simulink model "obstacleAvoidance"  (R2024b)
settings: Solver=VariableStepAuto  StartTime=0.0  StopTime=5  RelTol=1e-3
values from neighbouring files (symbols this model uses):
  TimeStep = 0.02    [obstacleAvoidance_data.sldd]
undefined symbols (not defined in the file or in its folder): driving, x0
libraries: drivingscenarioandsensors x2, simulink_extras x1
settings Model: DataDictionary=obstacleAvoidance_data.sldd  PacingRate=0.500000  Creator=kiwamoto  LastModifiedBy=tshintai
settings OptimizationCC: DefaultParameterBehavior=Inlined  EnhancedBackFolding=on  PassReuseOutputArgsAs=Individual arguments  ZeroExternalMemoryAtStartup=off  ZeroInternalMemoryAtStartup=off  OptimizeBlockOrder=speed  DifferentSizesBufferReuse=on  OptimizationCustomize=off  EfficientTunableParamExpr=on
settings DebuggingCC: ParameterTunabilityLossMsg=error  UnconnectedInputMsg=warning  UnconnectedOutputMsg=warning  UnconnectedLineMsg=warning
settings ModelReferenceCC: EnableRefExpFcnMdlSchedulingChecks=on
settings SFSimCC: MATLABDynamicMemAlloc=off
settings RTWCC: Description=Embedded Coder  SystemTargetFile=ert.tlc  TemplateMakefile=ert_default_tmf  CodeExecutionProfiling=on  CodeProfilingSaveOptions=AllData  GPUComputeCapability=3.5  DLArmComputeVersion=19.05
settings CodeAppCC: ForceParamTrailComments=on  IgnoreCustomStorageClasses=off  OperatorAnnotations=on  SimulinkDataObjDesc=on  SFDataObjDesc=on  InsertBlockDesc=on
settings ERTTargetCC: TargetLangStandard=C99 (ISO)  GenerateSampleERTMain=on  ERTCustomFileTemplate=example_file_process.tlc  DynamicArrayContainerType=coder::array

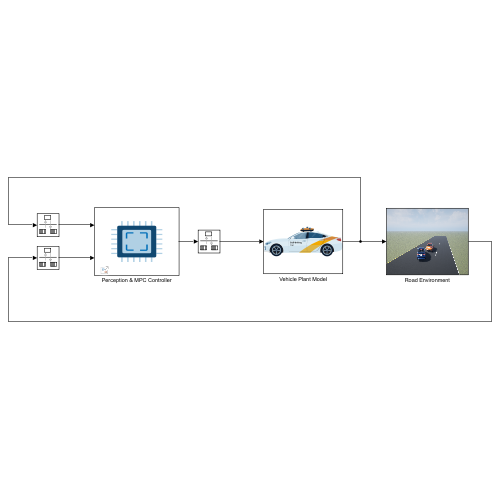
[thumbnail: Simulink's stored preview of the top-level diagram]
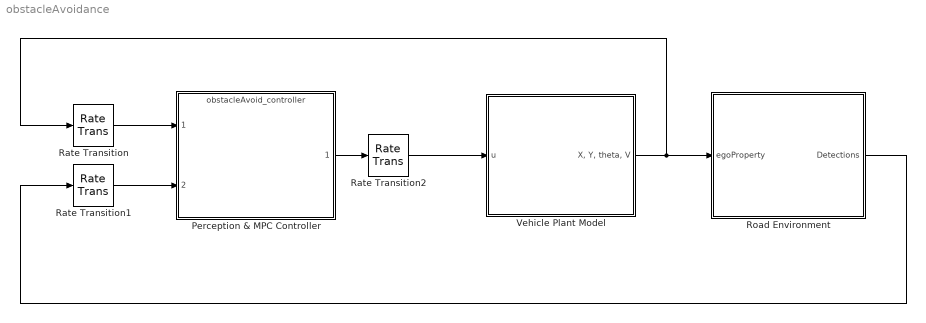
== system obstacleAvoidance ==
  Perception & MPC Controller : ModelReference  ModelNameDialog=obstacleAvoid_controller.slx  SimulationMode=Normal  ModelReferenceVersion=8.0
      mask Display: image('cpu-chip.svg'); % Use "Edit Image" on toolstrip to change.
  Rate Transition : RateTransition  OutPortSampleTime=TimeStep
  Rate Transition1 : RateTransition  OutPortSampleTime=TimeStep
  Rate Transition2 : RateTransition
  Road Environment : Subsystem
      mask Display: image('environment.PNG'); % Use "Edit Image" on toolstrip to change.
  Vehicle Plant Model : Subsystem
      mask Display: image('self-driving-car.svg'); % Use "Edit Image" on toolstrip to change.
  wires:
  Vehicle Plant Model/1("X, Y, theta, V") -> Rate Transition/1, Road Environment/1(egoProperty)
  Perception & MPC Controller/1 -> Rate Transition2/1
  Road Environment/1(Detections) -> Rate Transition1/1
  Rate Transition/1 -> Perception & MPC Controller/1
  Rate Transition1/1 -> Perception & MPC Controller/2
  Rate Transition2/1 -> Vehicle Plant Model/1(u)

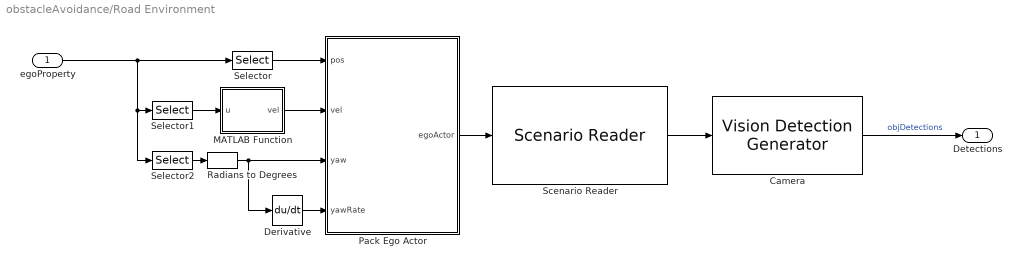
== system obstacleAvoidance/Road Environment ==
  egoProperty : Inport
  Camera : drivingscenarioandsensors/Vision Detection Generator  SensorIndex=1  DetectorOutput=Objects only  UpdateInterval=TimeStep  LaneUpdateInterval=TimeStep  SensorLocation=[3.7 0]  Height=1.1  Yaw=0  Pitch=0  Roll=0  BusNameSource=Auto  BusName=BusObjectDetections  BusName2Source=Auto  BusName2=BusLaneDetections  MaxNumDetectionsSource=Property  MaxNumDetections=1  MaxNumLanesSource=Property  MaxNumLanes=30  DetectionCoordinates=Sensor Cartesian  SimulateUsing=Interpreted execution  MaxRange=DetectionDistance  BoundingBoxAccuracy=10  ProcessNoiseIntensity=2  MaxSpeed=50  MaxAllowedOcclusion=0.2  MinObjectImageSize=[15 15]  DetectionProbability=1  FalsePositivesPerImage=0  MinLaneImageSize=[1 1]  LaneBoundaryAccuracy=1  HasNoise=off  InitialSeedSource=Repeatable  InitialSeed=0  UsedSeed=0  ActorProfilesSource=From Scenario Reader block  ActorProfilesParameters=driving.internal.ActorProfilesParameters  ActorProfilesExpression=[struct('ActorID',1,'ClassID',1,'Length',5,'Width',2,'Height',1.4,'OriginOffset',[-1.5 0 0],'MeshVertices',[4 1 0.857439446366782;4 -1 0.857439446366782;4 -1 0.314878892733564;4 1 0.314878892733564;4 1 0.857439446366782;2.75 1 0.993079584775086;2.75 -1 0.993079584775086;4 -1 0.857439446366782;2 0.8 1.4;0.5 0.8 1.4;0.5 -0.8 1.4;2 -0.8 1.4;-0.25 1 0.993079584775086;-1 1 0.857439446366782;-1 -1 0.857439446366782;-0.25 -1 0.993079584775086;4 1 0.857439446366782;4 1 0.314878892733564;2.75 1 0.314878892733564;2.75 1 0.993079584775086;2.75 1 0.993079584775086;2.75 1 0.314878892733564;-0.25 1 0.314878892733564;-0.25 1 0.993079584775086;-0.25 1 0.993079584775086;-0.25 1 0.314878892733564;-1 1 0.355570934256055;-1 1 0.857439446366782;2.75 1 0.993079584775086;-0.25 1 0.993079584775086;0.5 0.8 1.4;2 0.8 1.4;4 -1 0.857439446366782;4 -1 0.314878892733564;2.75 -1 0.314878892733564;2.75 -1 0.993079584775086;2.75 -1 0.993079584775086;2.75 -1 0.314878892733564;-0.25 -1 0.314878892733564;-0.25 -1 0.993079584775086;-0.25 -1 0.993079584775086;-0.25 -1 0.314878892733564;-1 -1 0.355570934256055;-1 -1 0.857439446366782;2.75 -1 0.993079584775086;-0.25 -1 0.993079584775086;0.5 -0.8 1.4;2 -0.8 1.4;-0.25 1 0.993079584775086;-0.25 -1 0.993079584775086;0.5 -0.8 1.4;0.5 0.8 1.4;2.75 -1 0.993079584775086;2 -0.8 1.4;2 0.8 1.4;2.75 1 0.993079584775086;-1 1 0.857439446366782;-1 1 0.355570934256055;-1 -1 0.355570934256055;-1 -1 0.857439446366782;4 1 0.314878892733564;4 -1 0.314878892733564;-0.25 -1 0.314878892733564;-0.25 1 0.314878892733564;-0.25 1 0.314878892733564;-1 1 0.355570934256055;-1 -1 0.355570934256055;-0.25 -1 0.314878892733564;0.0638297872340425 -0.7 0;0.0638297872340425 -0.966666666666667 0;0.267053411696866 -0.7 0.0601365173421445;0.267053411696866 -0.966666666666667 0.0601365173421445;0.392652518931835 -0.7 0.217575963708927;0.392652518931835 -0.966666666666667 0.217575963708927;0.392652518931835 -0.7 0.412181821758201;0.392652518931835 -0.966666666666667 0.412181821758201;0.267053411696866 -0.7 0.569621268124983;0.267053411696866 -0.966666666666667 0.569621268124983;0.0638297872340425 -0.7 0.629757785467128;0.0638297872340425 -0.966666666666667 0.629757785467128;-0.139393837228781 -0.7 0.569621268124983;-0.139393837228781 -0.966666666666667 0.569621268124983;-0.26499294446375 -0.7 0.412181821758201;-0.26499294446375 -0.966666666666667 0.412181821758201;-0.26499294446375 -0.7 0.217575963708927;-0.26499294446375 -0.966666666666667 0.217575963708927;-0.139393837228781 -0.7 0.0601365173421445;-0.139393837228781 -0.966666666666667 0.0601365173421445;0.0638297872340425 -0.7 0;0.0638297872340425 -0.966666666666667 0;0.0638297872340425 -0.7 0;0.267053411696866 -0.7 0.0601365173421445;0.392652518931835 -0.7 0.217575963708927;0.392652518931835 -0.7 0.412181821758201;0.267053411696866 -0.7 0.569621268124983;0.0638297872340425 -0.7 0.629757785467128;-0.139393837228781 -0.7 0.569621268124983;-0.26499294446375 -0.7 0.412181821758201;-0.26499294446375 -0.7 0.217575963708927;-0.139393837228781 -0.7 0.0601365173421445;0.0638297872340425 -0.966666666666667 0;0.267053411696866 -0.966666666666667 0.0601365173421445;0.392652518931835 -0.966666666666667 0.217575963708927;0.392652518931835 -0.966666666666667 0.412181821758201;0.267053411696866 -0.966666666666667 0.569621268124983;0.0638297872340425 -0.966666666666667 0.629757785467128;-0.139393837228781 -0.966666666666667 0.569621268124983;-0.26499294446375 -0.966666666666667 0.412181821758201;-0.26499294446375 -0.966666666666667 0.217575963708927;-0.139393837228781 -0.966666666666667 0.0601365173421445;0.0638297872340425 0.966666666666667 0;0.0638297872340425 0.7 0;0.267053411696866 0.966666666666667 0.0601365173421445;0.267053411696866 0.7 0.0601365173421445;0.392652518931835 0.966666666666667 0.217575963708927;0.392652518931835 0.7 0.217575963708927;0.392652518931835 0.966666666666667 0.412181821758201;0.392652518931835 0.7 0.412181821758201;0.267053411696866 0.966666666666667 0.569621268124983;0.267053411696866 0.7 0.569621268124983;0.0638297872340425 0.966666666666667 0.629757785467128;0.0638297872340425 0.7 ...(+5114 chars)],'MeshFaces',[1 2 3;3 4 1;5 6 7;7 8 5;9 10 11;11 12 9;13 14 15;15 16 13;17 18 19;19 20 17;21 22 23;23 24 21;25 26 27;27 28 25;29 30 31;31 32 29;33 34 35;35 36 33;37 38 39;39 40 37;41 42 43;43 44 41;45 46 47;47 48 45;49 50 51;51 52 49;53 54 55;55 56 53;57 58 59;59 60 57;61 62 63;63 64 61;65 66 67;67 68 65;69 71 72;72 70 69;71 73 74;74 72 71;73 75 76;76 74 73;75 77 78;78 76 75;77 79 80;80 78 77;79 81 82;82 80 79;81 83 84;84 82 81;83 85 86;86 84 83;85 87 88;88 86 85;87 89 90;90 88 87;91 92 93;91 93 94;91 94 95;91 95 96;91 96 97;91 97 98;91 98 99;91 99 100;101 102 103;101 103 104;101 104 105;101 105 106;101 106 107;101 107 108;101 108 109;101 109 110;111 113 114;114 112 111;113 115 116;116 114 113;115 117 118;118 116 115;117 119 120;120 118 117;119 121 122;122 120 119;121 123 124;124 122 121;123 125 126;126 124 123;125 127 128;128 126 125;127 129 130;130 128 127;129 131 132;132 130 129;133 134 135;133 135 136;133 136 137;133 137 138;133 138 139;133 139 140;133 140 141;133 141 142;143 144 145;143 145 146;143 146 147;143 147 148;143 148 149;143 149 150;143 150 151;143 151 152;153 155 156;156 154 153;155 157 158;158 156 155;157 159 160;160 158 157;159 161 162;162 160 159;161 163 164;164 162 161;163 165 166;166 164 163;165 167 168;168 166 165;167 169 170;170 168 167;169 171 172;172 170 169;171 173 174;174 172 171;175 176 177;175 177 178;175 178 179;175 179 180;175 180 181;175 181 182;175 182 183;175 183 184;185 186 187;185 187 188;185 188 189;185 189 190;185 190 191;185 191 192;185 192 193;185 193 194;195 197 198;198 196 195;197 199 200;200 198 197;199 201 202;202 200 199;201 203 204;204 202 201;203 205 206;206 204 203;205 207 208;208 206 205;207 209 210;210 208 207;209 211 212;212 210 209;211 213 214;214 212 211;213 215 216;216 214 213;217 218 219;217 219 220;217 220 221;217 221 222;217 222 223;217 223 224;217 224 225;217 225 226;227 228 229;227 229 230;227 230 231;227 231 232;227 232 233;227 233 234;227 234 235;227 235 236],'RCSPattern',[10 10;10 10],'RCSAzimuthAngles',[-180 180],'RCSElevationAngles',[-90 90]); struct('ActorID',2,'ClassID',1,'Length',5,'Width',2,'Height',1.4,'OriginOffset',[-1.5 0 0],'MeshVertices',[4 1 0.857439446366782;4 -1 0.857439446366782;4 -1 0.314878892733564;4 1 0.314878892733564;4 1 0.857439446366782;2.75 1 0.993079584775086;2.75 -1 0.993079584775086;4 -1 0.857439446366782;2 0.8 1.4;0.5 0.8 1.4;0.5 -0.8 1.4;2 -0.8 1.4;-0.25 1 0.993079584775086;-1 1 0.857439446366782;-1 -1 0.857439446366782;-0.25 -1 0.993079584775086;4 1 0.857439446366782;4 1 0.314878892733564;2.75 1 0.314878892733564;2.75 1 0.993079584775086;2.75 1 0.993079584775086;2.75 1 0.314878892733564;-0.25 1 0.314878892733564;-0.25 1 0.993079584775086;-0.25 1 0.993079584775086;-0.25 1 0.314878892733564;-1 1 0.355570934256055;-1 1 0.857439446366782;2.75 1 0.993079584775086;-0.25 1 0.993079584775086;0.5 0.8 1.4;2 0.8 1.4;4 -1 0.857439446366782;4 -1 0.314878892733564;2.75 -1 0.314878892733564;2.75 -1 0.993079584775086;2.75 -1 0.993079584775086;2.75 -1 0.314878892733564;-0.25 -1 0.314878892733564;-0.25 -1 0.993079584775086;-0.25 -1 0.993079584775086;-0.25 -1 0.314878892733564;-1 -1 0.355570934256055;-1 -1 0.857439446366782;2.75 -1 0.993079584775086;-0.25 -1 0.993079584775086;0.5 -0.8 1.4;2 -0.8 1.4;-0.25 1 0.993079584775086;-0.25 -1 0.993079584775086;0.5 -0.8 1.4;0.5 0.8 1.4;2.75 -1 0.993079584775086;2 -0.8 1.4;2 0.8 1.4;2.75 1 0.993079584775086;-1 1 0.857439446366782;-1 1 0.355570934256055;-1 -1 0.355570934256055;-1 -1 0.857439446366782;4 1 0.314878892733564;4 -1 0.314878892733564;-0.25 -1 0.314878892733564;-0.25 1 0.314878892733564;-0.25 1 0.314878892733564;-1 1 0.355570934256055;-1 -1 0.355570934256055;-0.25 -1 0.314878892733564;0.0638297872340425 -0.7 0;0.0638297872340425 -0.966666666666667 0;0.267053411696866 -0.7 0.0601365173421445;0.267053411696866 -0.966666666666667 0.0601365173421445;0.392652518931835 -0.7 0.217575963708927;0.392652518931835 -0.966666666666667 0.217575963708927;0.392652518931835 -0.7 0.412181821758201;0.392652518931835 -0.966666666666667 0.412181821758201;0.267053411696866 -0.7 0.569621268124983;0.267053411696866 -0.966666666666667 0.569621268124983;0.0638297872340425 -0.7 0.629757785467128;0.0638297872340425 -0.966666666666667 0.629757785467128;-0.139393837228781 -0.7 0.569621268124983;-0.139393837228781 -0.966666666666667 0.569621268124983;-0.26499294446375 -0.7 0.412181821758201;-0.26499294446375 -0.966666666666667 0.412181821758201;-0.26499294446375 -0.7 0.217575963708927;-0.26499294446375 -0.966666666666667 0.217575963708927;-0.139393837228781 -0.7 0.0601365173421445;-0.139393837228781 -0.966666666666667 0.0601365173421445;0.0638297872340425 -0.7 0;0.0638297872340425 -0.966666666666667 0;0.0638297872340425 -0.7 0;0.267053411696866 -0.7 0.0601365173421445;0.392652518931835 -0.7 0.217575963708927;0.392652518931835 -0.7 0.412181821758201;0.267053411696866 -0.7 0.569621268124983;0.0638297872340425 -0.7 0.629757785467128;-0.139393837228781 -0.7 0.569621268124983;-0.26499294446375 -0.7 0.412181821758201;-0.26499294446375 -0.7 0.217575963708927;-0.139393837228781 -0.7 0.0601365173421445;0.0638297872340425 -0.966666666666667 0;0.267053411696866 -0.966666666666667 0.0601365173421445;0.392652518931835 -0.966666666666667 0.217575963708927;0.392652518931835 -0.966666666666667 0.412181821758201;0.267053411696866 -0.966666666666667 0.569621268124983;0.0638297872340425 -0.966666666666667 0.629757785467128;-0.139393837228781 -0.966666666666667 0.569621268124983;-0.26499294446375 -0.966666666666667 0.412181821758201;-0.26499294446375 -0.966666666666667 0.217575963708927;-0.139393837228781 -0.966666666666667 0.0601365173421445;0.0638297872340425 0.966666666666667 0;0.0638297872340425 0.7 0;0.267053411696866 0.966666666666667 0.0601365173421445;0.267053411696866 0.7 0.0601365173421445;0.392652518931835 0.966666666666667 0.217575963708927;0.392652518931835 0.7 0.217575963708927;0.392652518931835 0.966666666666667 0.412181821758201;0.392652518931835 0.7 0.412181821758201;0.267053411696866 0.966666666666667 0.569621268124983;0.267053411696866 0.7 0.569621268124983;0.0638297872340425 0.966666666666667 0.629757785467128;0.0638297872340425 0.7 ...(+5114 chars)],'MeshFaces',[1 2 3;3 4 1;5 6 7;7 8 5;9 10 11;11 12 9;13 14 15;15 16 13;17 18 19;19 20 17;21 22 23;23 24 21;25 26 27;27 28 25;29 30 31;31 32 29;33 34 35;35 36 33;37 38 39;39 40 37;41 42 43;43 44 41;45 46 47;47 48 45;49 50 51;51 52 49;53 54 55;55 56 53;57 58 59;59 60 57;61 62 63;63 64 61;65 66 67;67 68 65;69 71 72;72 70 69;71 73 74;74 72 71;73 75 76;76 74 73;75 77 78;78 76 75;77 79 80;80 78 77;79 81 82;82 80 79;81 83 84;84 82 81;83 85 86;86 84 83;85 87 88;88 86 85;87 89 90;90 88 87;91 92 93;91 93 94;91 94 95;91 95 96;91 96 97;91 97 98;91 98 99;91 99 100;101 102 103;101 103 104;101 104 105;101 105 106;101 106 107;101 107 108;101 108 109;101 109 110;111 113 114;114 112 111;113 115 116;116 114 113;115 117 118;118 116 115;117 119 120;120 118 117;119 121 122;122 120 119;121 123 124;124 122 121;123 125 126;126 124 123;125 127 128;128 126 125;127 129 130;130 128 127;129 131 132;132 130 129;133 134 135;133 135 136;133 136 137;133 137 138;133 138 139;133 139 140;133 140 141;133 141 142;143 144 145;143 145 146;143 146 147;143 147 148;143 148 149;143 149 150;143 150 151;143 151 152;153 155 156;156 154 153;155 157 158;158 156 155;157 159 160;160 158 157;159 161 162;162 160 159;161 163 164;164 162 161;163 165 166;166 164 163;165 167 168;168 166 165;167 169 170;170 168 167;169 171 172;172 170 169;171 173 174;174 172 171;175 176 177;175 177 178;175 178 179;175 179 180;175 180 181;175 181 182;175 182 183;175 183 184;185 186 187;185 187 188;185 188 189;185 189 190;185 190 191;185 191 192;185 192 193;185 193 194;195 197 198;198 196 195;197 199 200;200 198 197;199 201 202;202 200 199;201 203 204;204 202 201;203 205 206;206 204 203;205 207 208;208 206 205;207 209 210;210 208 207;209 211 212;212 210 209;211 213 214;214 212 211;213 215 216;216 214 213;217 218 219;217 219 220;217 220 221;217 221 222;217 222 223;217 223 224;217 224 225;217 225 226;227 228 229;227 229 230;227 230 231;227 231 232;227 232 233;227 233 234;227 234 235;227 235 236],'RCSPattern',[10 10;10 10],'RCSAzimuthAngles',[-180 180],'RCSElevationAngles',[-90 90])]  Intrinsics=driving.internal.cameraIntrinsics('FocalLength',[800, 800],'PrincipalPoint',[320 240],'ImageSize',[580 1000],'RadialDistortion',[0 0],'TangentialDistortion',[0 0],'Skew',0)
  Derivative : Derivative
  MATLAB Function : MATLAB Function  TreatAsAtomicUnit=on
  Pack Ego Actor : MATLAB Function  TreatAsAtomicUnit=on
  Radians to Degrees : simulink_extras/Transformations/Radians to Degrees
  Scenario Reader : drivingscenarioandsensors/Scenario Reader  ScenarioSource=From file  ScenarioFileName=obstacleAvoidance_scenario.mat  ScenarioVariableName=scenario  OutputCoordinateSystem=Vehicle coordinates  EgoVehicleSource=Input port  EgoVehicleActorID=1  OrientVehiclesOnRoad=off  OutputEgoVehiclePose=off  OutputEgoVehicleState=off  SampleTime=TimeStep  LaneBoundaryOutput=None  LaneBoundaryDistance=0:0.5:9.5  LaneBoundaryLocation=Center of lane markings  BusNameSource=Auto  BusName=BusActorsActors  BusNumActorsSource=Scenario  BusNumActors=100  BusName2Source=Auto  BusName2=BusLaneBoundaries  BusNumLaneBoundariesSource=Scenario  BusNumLaneBoundaries=10  BusName3Source=Auto  BusName3=BusEgoActor  BusName4Source=Auto  BusName4=BusEgoState  ShowCoordinateLabels=on  SimulateUsing=Interpreted execution
  Selector : Selector  InputPortWidth=4  IndexOptions=Index vector (dialog)  Indices=[1 2]  OutputSizes=1
  Selector1 : Selector  InputPortWidth=4  IndexOptions=Index vector (dialog)  Indices=[3 4]  OutputSizes=1
  Selector2 : Selector  InputPortWidth=4  IndexOptions=Index vector (dialog)  Indices=3  OutputSizes=1
  Detections : Outport
  wires:
  MATLAB Function/1(vel) -> Pack Ego Actor/2(vel)
  Selector/1 -> Pack Ego Actor/1(pos)
  Derivative/1 -> Pack Ego Actor/4(yawRate)
  Selector1/1 -> MATLAB Function/1(u)
  Selector2/1 -> Radians to Degrees/1
  Pack Ego Actor/1(egoActor) -> Scenario Reader/1
  egoProperty/1 -> Selector2/1, Selector1/1, Selector/1
  Radians to Degrees/1 -> Derivative/1, Pack Ego Actor/3(yaw)
  Scenario Reader/1 -> Camera/1
  Camera/1 -> Detections/1  "objDetections"

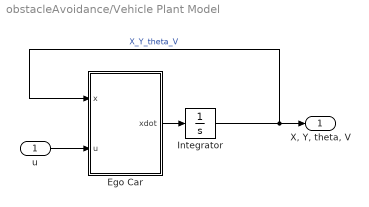
== system obstacleAvoidance/Vehicle Plant Model ==
  u : Inport
  Ego Car : MATLAB Function  TreatAsAtomicUnit=on
  Integrator : Integrator  InitialCondition=x0
  "X, Y, theta, V" : Outport
  wires:
  Integrator/1 -> Ego Car/1(x), "X, Y, theta, V"/1  "X_Y_theta_V"
  Ego Car/1(xdot) -> Integrator/1
  u/1 -> Ego Car/2(u)

== matlab function obstacleAvoidance/Road Environment/MATLAB Function ==
  data: u input size=2; vel output size=2
function vel = fcn(u)
theta = u(1);
V = u(2);
vel = zeros(2,1);

vel(1) = V*cos(theta);  %Vx
vel(2) = V*sin(theta);  %Vy

== matlab function obstacleAvoidance/Road Environment/Pack Ego Actor ==
  data: pos input; egoActor output Bus: BusActors1Actors size=1; vel input; yaw input; yawRate input
function egoActor = packEgo(pos,vel,yaw,yawRate)
% Pack ego information into a single ego actor bus
%
% Imoprtant note:
% Output is a bus of type BusActorsActors. This is the same bus used by the
% Scenario Reader to output an individual actor. If you change the
% output bus name of Scenario Reader, change the output bus name here
% as well by clicking on 'Edit Data' in the menu above.

egoActor = struct(...
    'ActorID',1,...
    'Position', [pos(1) pos(2) 0], ...
    'Velocity', [vel(1) vel(2) 0], ...
    'Roll', 0, ...
    'Pitch', 0, ...
    'Yaw', yaw, ...
    'AngularVelocity', [0 0 yawRate]);

== matlab function obstacleAvoidance/Vehicle Plant Model/Ego Car ==
  data: x input; u input; xdot output
function xdot = fcn(x,u)

xdot = obstacleVehicleModelCT(x,u);

end
